simulink model "Final_Simulation_BMWi3_Average_Model"  (R2021b)
settings: Solver=FixedStepAuto  StartTime=0.0  StopTime=10  FixedStep=Tsim  RelTol=1e-3
values from neighbouring files (symbols this model uses):
  A_front = 2.38    [parameters_BMWi3.m]
  C_drag = 0.29    [parameters_BMWi3.m]
  flux_mach = 200/(6*4800*pi/30)    (= 0.0663145596216)    [parameters_BMWi3.m]
  fr = 0.013    [parameters_BMWi3.m]
  id = I_demand .* cos(beta)    [parameters_BMWi3.m]
  Imotor_max = 400    [parameters_BMWi3.m]
  iq = I_demand .* sin(beta)    [parameters_BMWi3.m]
  J_mach = 0.0666    [parameters_BMWi3.m]
  k_gear = nmax_mach/nmax_wheel    (= 5.46098838726)    [parameters_BMWi3.m]
  Ki_id = Bw_c^2 * Ld_mach    (= 846.812057613)    [parameters_BMWi3.m]
  Ki_idc = 2*pi*BW_i*R_Lboost    (= 471.238898038)    [parameters_BMWi3.m]
  Ki_iq = Bw_c^2 * Lq_mach    (= 2368.70505626)    [parameters_BMWi3.m]
  Ki_vdc = Wn_v^2*C_boost    (= 84.3851176293)    [parameters_BMWi3.m]
  Kp_id = 2*xi_c*Bw_c*Ld_mach-R_phase_mach    [parameters_BMWi3.m]
  Kp_idc = 2*pi*BW_i*L_boost    (= 1.88495559215)    [parameters_BMWi3.m]
  Kp_iq = 2*xi_c*Bw_c*Lq_mach-R_phase_mach    [parameters_BMWi3.m]
  Kp_vdc = 2*xi*Wn_v*C_boost    [parameters_BMWi3.m]
  Ld_mach = 0.0858*1e-3    (= 8.58e-05)    [parameters_BMWi3.m]
  Lq_mach = 0.24*1e-3    (= 0.00024)    [parameters_BMWi3.m]
  mass = 1270    [parameters_BMWi3.m]
  p = 6    [parameters_BMWi3.m]
  r_wheel = (15+2*70/(100*175))*0.0254/2    (= 0.1906016)    [parameters_BMWi3.m]
  rho = 1.25    [parameters_BMWi3.m]
  T = zeros(1,length(w))    [parameters_BMWi3.m]
  T_dq = (3/2)*(p)*(flux_mach*iq+(Ld_mach-Lq_mach)*iq.*id)    [parameters_BMWi3.m]
  Tmax_mach = 250    [parameters_BMWi3.m]
  Tsim = 5e-6    (= 5e-06)    [parameters_BMWi3.m]
  Vdc = 600    [parameters_BMWi3.m]
  w = 0:1:Wmax    [parameters_BMWi3.m]
  wbase = Pmax*1e3/Tmax    (= 500)    [parameters_BMWi3.m]
undefined symbols (not defined in the file or in its folder): Ion, Lithium
libraries: nesl_utility x18, fl_lib x14, spsSecondOrderFilterLib x10, sdl_lib x8, slpidlib x7, spsMeanLib x6, simulink x4, ee_lib x4, simulink_extras x3, pid_lib x2, spsabctodq0Lib x1, drivingcycle_lib x1
(part 2 of 2)

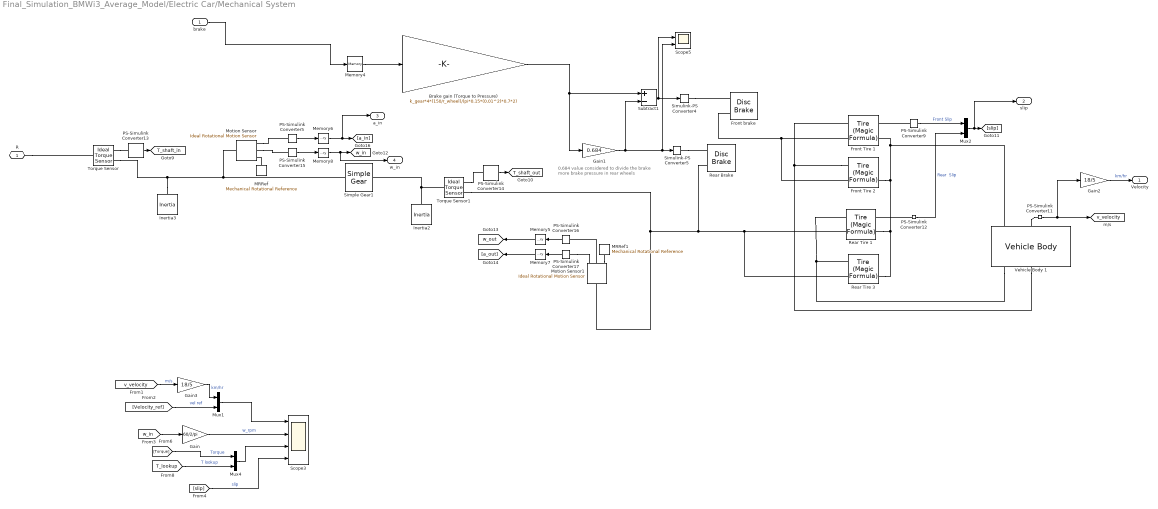
== system Final_Simulation_BMWi3_Average_Model/Electric Car/Mechanical System ==
  note: 0.684 value considered to divide the brake
      | more brake pressure in rear wheels
  brake : Inport
  " Rear Tire 1" : sdl_lib/Tires & Vehicles/Tire (Magic Formula)  parameterization=sdl.enum.magic_tire_model.peak  F_z1=3000 N  F_x1=3800 N  kappa1=10  B_m=10  C_m=1.9  D_m=1  E_m=0.97  fz0=4000 N  p_Cx=1.685  p_Dx=[1.21, -.037]  p_Ex=[.344, .095, -.02, 0]  p_Kx=[21.51, -.163, .245]  p_Hx=[-.002, .002]  p_Vx=[0, 0]  r_e=r_wheel m  model_compliance=sdl.enum.compliance.off  stiffness=1e6 N/m  damping=1000 N/(m/s)  model_inertia=sdl.enum.model_inertia.off  inertia=1 kg*m^2  initial_velocity=0 rad/s  model_resistance=simscape.enum.onoff.off  resistance_model=sdl.enum.rollingResistanceParameterization.velocity  coeff=0.015  p_tire=250e3 Pa  alpha=-0.003  beta=0.97  coeff_a=84e-4  coeff_b=6.2e-4 s/m  coeff_c=1.6e-4 s^2/m^2  v_thr=0.001 m/s  v_tr_thr=0.1 m/s
  Brake gain (Torque to Pressure) : Gain  Gain=k_gear*4*(150/r_wheel)/(pi*0.15*(0.01^2)*0.7*2)
  Front Tire 1 : sdl_lib/Tires & Vehicles/Tire (Magic Formula)  parameterization=sdl.enum.magic_tire_model.peak  F_z1=3000 N  F_x1=3800 N  kappa1=10  B_m=10  C_m=1.9  D_m=1  E_m=0.97  fz0=4000 N  p_Cx=1.685  p_Dx=[1.21, -.037]  p_Ex=[.344, .095, -.02, 0]  p_Kx=[21.51, -.163, .245]  p_Hx=[-.002, .002]  p_Vx=[0, 0]  r_e=r_wheel m  model_compliance=sdl.enum.compliance.off  stiffness=1e6 N/m  damping=1000 N/(m/s)  model_inertia=sdl.enum.model_inertia.off  inertia=1 kg*m^2  initial_velocity=0 rad/s  model_resistance=simscape.enum.onoff.off  resistance_model=sdl.enum.rollingResistanceParameterization.velocity  coeff=0.015  p_tire=250e3 Pa  alpha=-0.003  beta=0.97  coeff_a=84e-4  coeff_b=6.2e-4 s/m  coeff_c=1.6e-4 s^2/m^2  v_thr=0.001 m/s  v_tr_thr=0.1 m/s
  Front Tire 2 : sdl_lib/Tires & Vehicles/Tire (Magic Formula)  parameterization=sdl.enum.magic_tire_model.peak  F_z1=3000 N  F_x1=3800 N  kappa1=10  B_m=10  C_m=1.9  D_m=1  E_m=0.97  fz0=4000 N  p_Cx=1.685  p_Dx=[1.21, -.037]  p_Ex=[.344, .095, -.02, 0]  p_Kx=[21.51, -.163, .245]  p_Hx=[-.002, .002]  p_Vx=[0, 0]  r_e=r_wheel m  model_compliance=sdl.enum.compliance.off  stiffness=1e6 N/m  damping=1000 N/(m/s)  model_inertia=sdl.enum.model_inertia.off  inertia=1 kg*m^2  initial_velocity=0 rad/s  model_resistance=simscape.enum.onoff.off  resistance_model=sdl.enum.rollingResistanceParameterization.velocity  coeff=0.015  p_tire=250e3 Pa  alpha=-0.003  beta=0.97  coeff_a=84e-4  coeff_b=6.2e-4 s/m  coeff_c=1.6e-4 s^2/m^2  v_thr=0.001 m/s  v_tr_thr=0.1 m/s
  Front brake : sdl_lib/Brakes & Detents/Rotational/Disc Brake  r_mean=150 mm  bore=10 mm  n_pads=2  thermal_port=simscape.enum.thermaleffects.omit  mu_static=0.9  mu_coulomb=0.7  temperature_TLU=[280, 300, 320] K  mu_static_TLU=[.9, .8, .7]  mu_coulomb_TLU=[.8, .7, .6]  brkwy_vel=0.1 rad/s  visc_coef=.001 N*m/(rad/s)  enable_faults=simscape.enum.onoff.off  faulted_pressure=0 bar  external_fault=simscape.enum.onoff.off  temporal_fault=simscape.enum.onoff.off  fault_time=5 s  report_fault=simscape.enum.assert.action.none  thermal_mass=50 kJ/K  temperature_specify=off  temperature_priority=High  temperature=300 K  temperature_nominal_specify=off  temperature_nominal_unit=K  temperature_nominal_value=1
      settings: SourceProductBaseCode=LD
  Gain : Gain  Gain=60/2/pi
  Gain1 : Gain  Gain=0.684
  Gain2 : Gain  Gain=18/5
  Gain3 : Gain  Gain=18/5
  Inertia2 : fl_lib/Mechanical/Rotational Elements/Inertia  inertia=J_mach kg*m^2  num_ports=foundation.enum.numPorts2.one  w_specify=off  w_priority=High  w=0 rad/s  w_nominal_specify=off  w_nominal_unit=rad/s  w_nominal_value=1  t_specify=off  t_priority=None  t=0 N*m  t_nominal_specify=off  t_nominal_unit=N*m  t_nominal_value=1
  Inertia3 : fl_lib/Mechanical/Rotational Elements/Inertia  inertia=J_mach kg*m^2  num_ports=foundation.enum.numPorts2.one  w_specify=off  w_priority=High  w=0 rad/s  w_nominal_specify=off  w_nominal_unit=rad/s  w_nominal_value=1  t_specify=off  t_priority=None  t=0 N*m  t_nominal_specify=off  t_nominal_unit=N*m  t_nominal_value=1
  MRRef : fl_lib/Mechanical/Rotational Elements/Mechanical Rotational Reference
      settings: SourceProductName=Foundation Library
  MRRef1 : fl_lib/Mechanical/Rotational Elements/Mechanical Rotational Reference
      settings: SourceProductName=Foundation Library
  Memory{4..8} (5 alike) : Memory
  Motion Sensor : fl_lib/Mechanical/Mechanical Sensors/Ideal Rotational Motion Sensor  wrap_angle=simscape.enum.onoff.off  offset=0 rad
      settings: SourceProductName=Foundation Library
  Motion Sensor1 : fl_lib/Mechanical/Mechanical Sensors/Ideal Rotational Motion Sensor  wrap_angle=simscape.enum.onoff.off  offset=0 rad
      settings: SourceProductName=Foundation Library
  Mux1 : Mux  Inputs=2
  Mux2 : Mux  Inputs=2
  Mux4 : Mux  Inputs=2
  PS-Simulink Converter{5,9,11..12,15..17} (7 alike) : nesl_utility/PS-Simulink Converter  PhysicalDomain=network_engine_domain  SubClassName=ps_output  LeftPortType=input  RightPortType=output  PseudoPeriodic=off  Frequencies=[]  Unit=inherit  AffineConversion=off
      PS-Simulink Converter15 settings: SourceProductBaseCode=PW,SS
      PS-Simulink Converter16 settings: SourceProductBaseCode=PW,SS
      PS-Simulink Converter17 settings: SourceProductBaseCode=PW,SS
      PS-Simulink Converter5 settings: SourceProductBaseCode=PW,SS
  PS-Simulink Converter13 : nesl_utility/PS-Simulink Converter  PhysicalDomain=network_engine_domain  SubClassName=ps_output  LeftPortType=input  RightPortType=output  PseudoPeriodic=off  Frequencies=[]  Unit=N*m  AffineConversion=off
      settings: SourceProductName=Utilities
  PS-Simulink Converter14 : nesl_utility/PS-Simulink Converter  PhysicalDomain=network_engine_domain  SubClassName=ps_output  LeftPortType=input  RightPortType=output  PseudoPeriodic=off  Frequencies=[]  Unit=N*m  AffineConversion=off
      settings: SourceProductName=Utilities
  Rear Brake : sdl_lib/Brakes & Detents/Rotational/Disc Brake  r_mean=150 mm  bore=10 mm  n_pads=2  thermal_port=simscape.enum.thermaleffects.omit  mu_static=0.9  mu_coulomb=0.7  temperature_TLU=[280, 300, 320] K  mu_static_TLU=[.9, .8, .7]  mu_coulomb_TLU=[.8, .7, .6]  brkwy_vel=0.1 rad/s  visc_coef=.001 N*m/(rad/s)  enable_faults=simscape.enum.onoff.off  faulted_pressure=0 bar  external_fault=simscape.enum.onoff.off  temporal_fault=simscape.enum.onoff.off  fault_time=5 s  report_fault=simscape.enum.assert.action.none  thermal_mass=50 kJ/K  temperature_specify=off  temperature_priority=High  temperature=300 K  temperature_nominal_specify=off  temperature_nominal_unit=K  temperature_nominal_value=1
      settings: SourceProductBaseCode=LD
  Rear Tire 3 : sdl_lib/Tires & Vehicles/Tire (Magic Formula)  parameterization=sdl.enum.magic_tire_model.peak  F_z1=3000 N  F_x1=3800 N  kappa1=10  B_m=10  C_m=1.9  D_m=1  E_m=0.97  fz0=4000 N  p_Cx=1.685  p_Dx=[1.21, -.037]  p_Ex=[.344, .095, -.02, 0]  p_Kx=[21.51, -.163, .245]  p_Hx=[-.002, .002]  p_Vx=[0, 0]  r_e=r_wheel m  model_compliance=sdl.enum.compliance.off  stiffness=1e6 N/m  damping=1000 N/(m/s)  model_inertia=sdl.enum.model_inertia.off  inertia=1 kg*m^2  initial_velocity=0 rad/s  model_resistance=simscape.enum.onoff.off  resistance_model=sdl.enum.rollingResistanceParameterization.velocity  coeff=0.015  p_tire=250e3 Pa  alpha=-0.003  beta=0.97  coeff_a=84e-4  coeff_b=6.2e-4 s/m  coeff_c=1.6e-4 s^2/m^2  v_thr=0.001 m/s  v_tr_thr=0.1 m/s
  Scope3 : Scope  NumInputPorts=4
  Scope5 : Scope  NumInputPorts=2
  Simple Gear1 : sdl_lib/Gears/Simple Gear  ratio=k_gear  rotation_direction=sdl.enum.shaftOutputDirection.same  friction_model=sdl.enum.gear_efficiencies_load.off  T_noload=0.1 N*m  T_nom=5 N*m  efficiency_nom=0.8  efficiency=0.8  temperature_TLU=[280, 300, 320] K  load_TLU=[1, 5, 10] N*m  efficiency_TLU=[.95, .9, .85]  efficiency_TLU2=[.85, .8, .75; .95, .9, .85; .85, .8, .7]  w_thr=0.01 rad/s  pwr_thr=0.001 W  backlash_model=sdl.enum.backlashModel.Off  backlash_distance=1e-3 mm  x0=0 mm  r_base=0.1 m  hardstop_model=simscape.enum.hardstop.smooth  transition=1e-4 mm  backlash_stiffness=1e7 N/m  backlash_damping=1e6 N/(m/s)  e=0  v_tol=0.001 m/s  mu_visc=[0, 0] N*m/(rad/s)  enable_faults=simscape.enum.onoff.off  efficiency_fault=0.05  external_fault=simscape.enum.onoff.off  temporal_fault=simscape.enum.onoff.off  fault_time=5 s  fault_angles=pi / 12 rad  report_fault=simscape.enum.assert.action.none  thermal_mass=50 J/K  temperature_specify=off  temperature_priority=High  temperature=300 K  temperature_nominal_specify=off  temperature_nominal_unit=K  temperature_nominal_value=1  x_backlash_specify=off  x_backlash_priority=None  x_backlash=0 mm  x_backlash_nominal_specify=off  x_backlash_nominal_unit=mm  x_backlash_nominal_value=1  f_hardstop_specify=off  f_hardstop_priority=None  f_hardstop=0 N  f_hardstop_nominal_specify=off  f_hardstop_nominal_unit=N  f_hardstop_nominal_value=1  v_backlash_specify=off  v_backlash_priority=None  v_backlash=0 m/s  v_backlash_nominal_specify=off  v_backlash_nominal_unit=m/s  v_backlash_nominal_value=1
  Simulink-PS Converter4 : nesl_utility/Simulink-PS Converter  PhysicalDomain=network_engine_domain  SubClassName=ps_input  LeftPortType=input  RightPortType=output  PseudoPeriodic=off  Frequencies=[]  NoiseDistribution=none  NoiseParameters=[]  Unit=Pa  AffineConversion=off  FilteringAndDerivatives=provide  SimscapeFilterOrder=1  InputFilterTimeConstant=0.001  UdotUserProvided=0
  Simulink-PS Converter5 : nesl_utility/Simulink-PS Converter  PhysicalDomain=network_engine_domain  SubClassName=ps_input  LeftPortType=input  RightPortType=output  PseudoPeriodic=off  Frequencies=[]  NoiseDistribution=none  NoiseParameters=[]  Unit=Pa  AffineConversion=off  FilteringAndDerivatives=provide  SimscapeFilterOrder=1  InputFilterTimeConstant=0.001  UdotUserProvided=0
  Subtract1 : Sum  Inputs=+-
  Torque Sensor : fl_lib/Mechanical/Mechanical Sensors/Ideal Torque Sensor
      settings: SourceProductName=Foundation Library
  Torque Sensor1 : fl_lib/Mechanical/Mechanical Sensors/Ideal Torque Sensor
      settings: SourceProductName=Foundation Library
  Vehicle Body 1 : sdl_lib/Tires & Vehicles/Vehicle Body  mass=mass kg  n_w=2  x_f=1.2 m  x_r=1.37 m  y_c=CoG_z m  mass_var=simscape.enum.onoff.off  g=9.81 m/s^2  liftoff_warning=simscape.enum.onoff.off  area=A_front m^2  Cd=C_drag  rho=1.18 kg/m^3  model_pitch=simscape.enum.onoff.off  inertia=4000 kg*m^2  suspension_model=sdl.enum.linearTLU.linear  k_f=1e4 N/m  b_f=1e4 N/(m/s)  k_r=1e4 N/m  b_r=1e4 N/(m/s)  k_f_TLU=[-2000, -1000, 0, 1000, 2000] N  x_f_TLU=[-.4, -.2, 0, .2, .4] m  b_f_TLU=[-200, -100, 0, 100, 200] N  v_f_TLU=[-4, -2, 0, 2, 4] m/s  k_r_TLU=[-2000, -1000, 0, 1000, 2000] N  x_r_TLU=[-.4, -.2, 0, .2, .4] m  b_r_TLU=[-200, -100, 0, 100, 200] N  v_r_TLU=[-4, -2, 0, 2, 4] m/s  interp_method=simscape.enum.interpolation.linear  extrap_method=simscape.enum.extrapolation.linear  model_hardstop=simscape.enum.onoff.off  upper_bound_f=.25 m  lower_bound_f=-.25 m  stop_k_f=1e6 N/m  stop_b_f=150 N/(m/s)  upper_bound_r=.25 m  lower_bound_r=-.25 m  stop_k_r=1e6 N/m  stop_b_r=150 N/(m/s)  initial_pitch=0 rad  initial_pitch_rate=0 rad/s  v_specify=off  v_priority=High  v=0 m/s  v_nominal_specify=off  v_nominal_unit=m/s  v_nominal_value=1
  R : PMIOPort  Side=Left
  Velocity : Outport
  slip : Outport  Port=2
  a_in : Outport  Port=3
  w_in : Outport  Port=4
  tag scope: T_shaft_in=global, T_shaft_out=global, v_velocity=global, w_in=global, w_out=global
  wires:
  PS-Simulink Converter17/1 -> Memory7/1
  Memory8/1 -> w_in/1, [w_in]
  [w_in] -> Gain/1
  PS-Simulink Converter13/1 -> [T_shaft_in]
  [Velocity_ref] -> Mux1/2  "vel ref"
  PS-Simulink Converter16/1 -> Memory5/1
  PS-Simulink Converter9/1 -> Mux2/1  "Front Slip"
  PS-Simulink Converter5/1 -> Memory6/1
  Gain/1 -> Scope3/2  "w_rpm"
  PS-Simulink Converter15/1 -> Memory8/1
  Memory7/1 -> [a_out]
  Memory5/1 -> [w_out]
  [T_lookup] -> Mux4/2  "T lookup"
  Memory4/1 -> Brake gain (Torque to Pressure)/1
  Subtract1/1 -> Scope5/1, Simulink-PS Converter4/1
  Memory6/1 -> a_in/1, [a_in]
  Brake gain (Torque to Pressure)/1 -> Gain1/1, Subtract1/1
  Mux2/1 -> slip/1, [slip]
  [Torque] -> Mux4/1  "Torque"
  PS-Simulink Converter12/1 -> Mux2/2  "Rear  Slip"
  [v_velocity] -> Gain3/1  "m/s"
  [slip] -> Scope3/4  "slip"
  Gain1/1 -> Simulink-PS Converter5/1, Scope5/2, Subtract1/2
  Gain3/1 -> Mux1/1  "km/hr"
  PS-Simulink Converter14/1 -> [T_shaft_out]
  Mux4/1 -> Scope3/3
  Mux1/1 -> Scope3/1
  PS-Simulink Converter11/1 -> Gain2/1, [v_velocity]
  brake/1 -> Memory4/1
  Gain2/1 -> Velocity/1  "km/hr"
  connections:
  Front Tire 2/LConn1 -- Vehicle Body 1/RConn2 -- Front Tire 1/LConn1
  Front Tire 2/RConn2 -- Rear Tire 3/RConn2 -- " Rear Tire 1"/RConn2 -- Front Tire 1/RConn2 -- Vehicle Body 1/LConn1
  Motion Sensor1/LConn1 -- Rear Brake/LConn2 -- " Rear Tire 1"/LConn2 -- Rear Tire 3/LConn2 -- Torque Sensor1/RConn1
  Front Tire 1/LConn2 -- Front Tire 2/LConn2 -- Front brake/LConn2
  Torque Sensor1/LConn1 -- Inertia2/LConn1 -- Simple Gear1/RConn1
  " Rear Tire 1"/LConn1 -- Vehicle Body 1/RConn1 -- Rear Tire 3/LConn1
  Inertia3/LConn1 -- Simple Gear1/LConn1 -- Motion Sensor/LConn1 -- Torque Sensor/RConn1
  Motion Sensor1/RConn2 -- PS-Simulink Converter16/LConn1
  Motion Sensor/RConn2 -- PS-Simulink Converter15/LConn1
  PS-Simulink Converter17/LConn1 -- Motion Sensor1/RConn3
  MRRef/LConn1 -- Motion Sensor/RConn1
  Motion Sensor/RConn3 -- PS-Simulink Converter5/LConn1
  Simulink-PS Converter5/RConn1 -- Rear Brake/LConn1
  Torque Sensor1/RConn2 -- PS-Simulink Converter14/LConn1
  MRRef1/LConn1 -- Motion Sensor1/RConn1
  Torque Sensor/RConn2 -- PS-Simulink Converter13/LConn1
  Vehicle Body 1/LConn2 -- PS-Simulink Converter11/LConn1
  Simulink-PS Converter4/RConn1 -- Front brake/LConn1
  PS-Simulink Converter9/LConn1 -- Front Tire 1/RConn1
  PS-Simulink Converter12/LConn1 -- " Rear Tire 1"/RConn1
  R/RConn1 -- Torque Sensor/LConn1

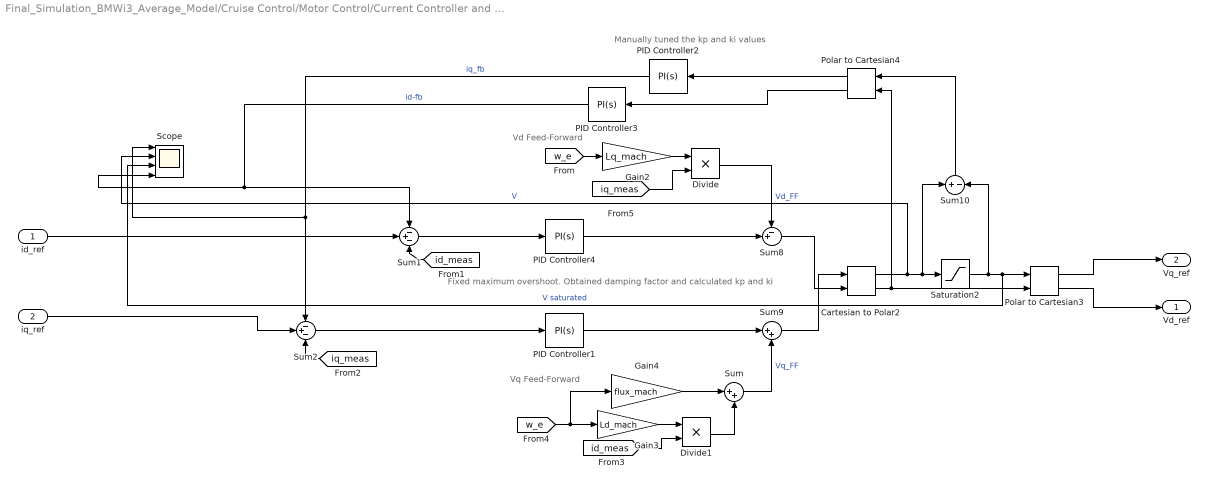
== system Final_Simulation_BMWi3_Average_Model/Cruise Control/Motor Control/Current Controller and Field Weakening ==
  note: Manually tuned the kp and ki values
  note: Fixed maximum overshoot. Obtained damping factor and calculated kp and ki
  note: Vd Feed-Forward
  note: Vq Feed-Forward
  id_ref : Inport
  iq_ref : Inport  Port=2
  Cartesian to Polar2 : simulink_extras/Transformations/Cartesian to Polar
  Divide : Product  Inputs=**
  Divide1 : Product  Inputs=**
  Gain2 : Gain  Gain=Lq_mach
  Gain3 : Gain  Gain=Ld_mach
  Gain4 : Gain  Gain=flux_mach
  PID Controller1 : slpidlib/PID Controller  Controller=PI  Form=Parallel  TimeDomain=Continuous-time  UseExternalTs=off  SampleTime=-1  IntegratorMethod=Forward Euler  FilterMethod=Forward Euler  ControllerParametersSource=internal  P=Kp_iq*1.4  I=Ki_iq*0.9  D=0  UseFilter=on  N=100  TunerSelectOption=Transfer Function Based (PID Tuner App)  InitialConditionSource=internal  InitialConditionForIntegrator=0  InitialConditionForFilter=0  DifferentiatorICPrevScaledInput=0  ExternalReset=none  TrackingMode=off  Kt=1  LimitOutput=on  SatLimitsSource=internal  UpperSaturationLimit=Vdc/sqrt(3)/sqrt(2)  LowerSaturationLimit=-Vdc/sqrt(3)/sqrt(2)  LinearizeAsGain=off  AntiWindupMode=clamping  Kb=1  POutMin=[]  POutMax=[]  IOutMin=[]  IOutMax=[]  DOutMin=[]  DOutMax=[]  NOutMin=[]  NOutMax=[]  SumOutMin=[]  SumOutMax=[]  SaturationOutMin=[]  SaturationOutMax=[]  PParamMin=[]  PParamMax=[]  IParamMin=[]  IParamMax=[]  DParamMin=[]  DParamMax=[]  NParamMin=[]  NParamMax=[]  KbParamMin=[]  KbParamMax=[]  KtParamMin=[]  KtParamMax=[]  KbOutMin=[]  KbOutMax=[]  KtOutMin=[]  KtOutMax=[]  IntegratorOutMin=[]  IntegratorOutMax=[]  FilterOutMin=[]  FilterOutMax=[]  SumI1OutMin=[]  SumI1OutMax=[]  SumI2OutMin=[]  SumI2OutMax=[]  SumI3OutMin=[]  SumI3OutMax=[]  SumI4OutMin=[]  SumI4OutMax=[]  SumDOutMin=[]  SumDOutMax=[]  DifferentiatorOutMin=[]  DifferentiatorOutMax=[]  FilterDiffOutCoefMin=[]  FilterDiffOutCoefMax=[]  ReciprocalOutMin=[]  ReciprocalOutMax=[]  SumDenOutMin=[]  SumDenOutMax=[]  SumNumOutMin=[]  SumNumOutMax=[]  DivideOutMin=[]  DivideOutMax=[]  UdiffTsProdOutMin=[]  UdiffTsProdOutMax=[]  NTsProdOutMin=[]  NTsProdOutMax=[]  UintegralTsProdOutMin=[]  UintegralTsProdOutMax=[]  UngainTsProdOutMin=[]  UngainTsProdOutMax=[]  IntegratorContinuousStateAttributes=''  IntegratorStateMustResolveToSignalObject=off  IntegratorRTWStateStorageClass=Auto  FilterContinuousStateAttributes=''  FilterStateMustResolveToSignalObject=off  FilterRTWStateStorageClass=Auto  ParallelPVariant=InternalParameters  IdealPVariant=Disabled  IVariant=InternalParameters  DVariant=Disabled  IntegratorVariant=Continuous  SatVariant=Enabled  AWVariant=ContClampingParallel  PCopyVariant=Disabled  TRVariant=Disabled  FdbkBlocksVariant=Forward  IdealPFdbkVariant=Disabled  SatFdbkVariant=Disabled  DerivativeFilterVariant=Disabled  NVariant=Disabled  NCopyVariant=Disabled_SignalSpec  FilterICVariant=Disabled  IntegratorICVariant=InternalICs  ExternalResetVariant=Disabled  TRSumVariant=Passthrough  SumFdbkVariant=Disabled  SumVariant=Sum_PI  TsampFilterVariant=InternalTs  TsampNgainVariant=Passthrough  TsampIntegralVariant=Passthrough  ExternalSaturationOutDataTypeStr=Inherit: Same as second input
  PID Controller2 : slpidlib/PID Controller  Controller=PI  Form=Parallel  TimeDomain=Continuous-time  UseExternalTs=off  SampleTime=-1  IntegratorMethod=Forward Euler  FilterMethod=Forward Euler  ControllerParametersSource=internal  P=0.8  I=75  D=0  UseFilter=on  N=100  TunerSelectOption=Transfer Function Based (PID Tuner App)  InitialConditionSource=internal  InitialConditionForIntegrator=0  InitialConditionForFilter=0  DifferentiatorICPrevScaledInput=0  ExternalReset=none  TrackingMode=off  Kt=1  LimitOutput=on  SatLimitsSource=internal  UpperSaturationLimit=Imotor_max  LowerSaturationLimit=-Imotor_max  LinearizeAsGain=on  AntiWindupMode=none  Kb=1  POutMin=[]  POutMax=[]  IOutMin=[]  IOutMax=[]  DOutMin=[]  DOutMax=[]  NOutMin=[]  NOutMax=[]  SumOutMin=[]  SumOutMax=[]  SaturationOutMin=[]  SaturationOutMax=[]  PParamMin=[]  PParamMax=[]  IParamMin=[]  IParamMax=[]  DParamMin=[]  DParamMax=[]  NParamMin=[]  NParamMax=[]  KbParamMin=[]  KbParamMax=[]  KtParamMin=[]  KtParamMax=[]  KbOutMin=[]  KbOutMax=[]  KtOutMin=[]  KtOutMax=[]  IntegratorOutMin=[]  IntegratorOutMax=[]  FilterOutMin=[]  FilterOutMax=[]  SumI1OutMin=[]  SumI1OutMax=[]  SumI2OutMin=[]  SumI2OutMax=[]  SumI3OutMin=[]  SumI3OutMax=[]  SumI4OutMin=[]  SumI4OutMax=[]  SumDOutMin=[]  SumDOutMax=[]  DifferentiatorOutMin=[]  DifferentiatorOutMax=[]  FilterDiffOutCoefMin=[]  FilterDiffOutCoefMax=[]  ReciprocalOutMin=[]  ReciprocalOutMax=[]  SumDenOutMin=[]  SumDenOutMax=[]  SumNumOutMin=[]  SumNumOutMax=[]  DivideOutMin=[]  DivideOutMax=[]  UdiffTsProdOutMin=[]  UdiffTsProdOutMax=[]  NTsProdOutMin=[]  NTsProdOutMax=[]  UintegralTsProdOutMin=[]  UintegralTsProdOutMax=[]  UngainTsProdOutMin=[]  UngainTsProdOutMax=[]  IntegratorContinuousStateAttributes=''  IntegratorStateMustResolveToSignalObject=off  IntegratorRTWStateStorageClass=Auto  FilterContinuousStateAttributes=''  FilterStateMustResolveToSignalObject=off  FilterRTWStateStorageClass=Auto  ParallelPVariant=InternalParameters  IdealPVariant=Disabled  IVariant=InternalParameters  DVariant=Disabled  IntegratorVariant=Continuous  SatVariant=Enabled  AWVariant=Passthrough  PCopyVariant=Disabled  TRVariant=Disabled  FdbkBlocksVariant=Forward  IdealPFdbkVariant=Disabled  SatFdbkVariant=Disabled  DerivativeFilterVariant=Disabled  NVariant=Disabled  NCopyVariant=Disabled_SignalSpec  FilterICVariant=Disabled  IntegratorICVariant=InternalICs  ExternalResetVariant=Disabled  TRSumVariant=Passthrough  SumFdbkVariant=Disabled  SumVariant=Sum_PI  TsampFilterVariant=InternalTs  TsampNgainVariant=Passthrough  TsampIntegralVariant=Passthrough  ExternalSaturationOutDataTypeStr=Inherit: Same as second input
  PID Controller3 : slpidlib/PID Controller  Controller=PI  Form=Parallel  TimeDomain=Continuous-time  UseExternalTs=off  SampleTime=-1  IntegratorMethod=Forward Euler  FilterMethod=Forward Euler  ControllerParametersSource=internal  P=0.9  I=-10  D=0  UseFilter=on  N=100  TunerSelectOption=Transfer Function Based (PID Tuner App)  InitialConditionSource=internal  InitialConditionForIntegrator=0  InitialConditionForFilter=0  DifferentiatorICPrevScaledInput=0  ExternalReset=none  TrackingMode=off  Kt=1  LimitOutput=on  SatLimitsSource=internal  UpperSaturationLimit=Imotor_max/4  LowerSaturationLimit=-Imotor_max/4  LinearizeAsGain=on  AntiWindupMode=none  Kb=1  POutMin=[]  POutMax=[]  IOutMin=[]  IOutMax=[]  DOutMin=[]  DOutMax=[]  NOutMin=[]  NOutMax=[]  SumOutMin=[]  SumOutMax=[]  SaturationOutMin=[]  SaturationOutMax=[]  PParamMin=[]  PParamMax=[]  IParamMin=[]  IParamMax=[]  DParamMin=[]  DParamMax=[]  NParamMin=[]  NParamMax=[]  KbParamMin=[]  KbParamMax=[]  KtParamMin=[]  KtParamMax=[]  KbOutMin=[]  KbOutMax=[]  KtOutMin=[]  KtOutMax=[]  IntegratorOutMin=[]  IntegratorOutMax=[]  FilterOutMin=[]  FilterOutMax=[]  SumI1OutMin=[]  SumI1OutMax=[]  SumI2OutMin=[]  SumI2OutMax=[]  SumI3OutMin=[]  SumI3OutMax=[]  SumI4OutMin=[]  SumI4OutMax=[]  SumDOutMin=[]  SumDOutMax=[]  DifferentiatorOutMin=[]  DifferentiatorOutMax=[]  FilterDiffOutCoefMin=[]  FilterDiffOutCoefMax=[]  ReciprocalOutMin=[]  ReciprocalOutMax=[]  SumDenOutMin=[]  SumDenOutMax=[]  SumNumOutMin=[]  SumNumOutMax=[]  DivideOutMin=[]  DivideOutMax=[]  UdiffTsProdOutMin=[]  UdiffTsProdOutMax=[]  NTsProdOutMin=[]  NTsProdOutMax=[]  UintegralTsProdOutMin=[]  UintegralTsProdOutMax=[]  UngainTsProdOutMin=[]  UngainTsProdOutMax=[]  IntegratorContinuousStateAttributes=''  IntegratorStateMustResolveToSignalObject=off  IntegratorRTWStateStorageClass=Auto  FilterContinuousStateAttributes=''  FilterStateMustResolveToSignalObject=off  FilterRTWStateStorageClass=Auto  ParallelPVariant=InternalParameters  IdealPVariant=Disabled  IVariant=InternalParameters  DVariant=Disabled  IntegratorVariant=Continuous  SatVariant=Enabled  AWVariant=Passthrough  PCopyVariant=Disabled  TRVariant=Disabled  FdbkBlocksVariant=Forward  IdealPFdbkVariant=Disabled  SatFdbkVariant=Disabled  DerivativeFilterVariant=Disabled  NVariant=Disabled  NCopyVariant=Disabled_SignalSpec  FilterICVariant=Disabled  IntegratorICVariant=InternalICs  ExternalResetVariant=Disabled  TRSumVariant=Passthrough  SumFdbkVariant=Disabled  SumVariant=Sum_PI  TsampFilterVariant=InternalTs  TsampNgainVariant=Passthrough  TsampIntegralVariant=Passthrough  ExternalSaturationOutDataTypeStr=Inherit: Same as second input
  PID Controller4 : slpidlib/PID Controller  Controller=PI  Form=Parallel  TimeDomain=Continuous-time  UseExternalTs=off  SampleTime=-1  IntegratorMethod=Forward Euler  FilterMethod=Forward Euler  ControllerParametersSource=internal  P=Kp_id*1.3  I=Ki_id*0.9  D=0  UseFilter=on  N=100  TunerSelectOption=Transfer Function Based (PID Tuner App)  InitialConditionSource=internal  InitialConditionForIntegrator=0  InitialConditionForFilter=0  DifferentiatorICPrevScaledInput=0  ExternalReset=none  TrackingMode=off  Kt=1  LimitOutput=on  SatLimitsSource=internal  UpperSaturationLimit=Vdc/sqrt(3)/sqrt(2)  LowerSaturationLimit=-Vdc/sqrt(3)/sqrt(2)  LinearizeAsGain=off  AntiWindupMode=clamping  Kb=1  POutMin=[]  POutMax=[]  IOutMin=[]  IOutMax=[]  DOutMin=[]  DOutMax=[]  NOutMin=[]  NOutMax=[]  SumOutMin=[]  SumOutMax=[]  SaturationOutMin=[]  SaturationOutMax=[]  PParamMin=[]  PParamMax=[]  IParamMin=[]  IParamMax=[]  DParamMin=[]  DParamMax=[]  NParamMin=[]  NParamMax=[]  KbParamMin=[]  KbParamMax=[]  KtParamMin=[]  KtParamMax=[]  KbOutMin=[]  KbOutMax=[]  KtOutMin=[]  KtOutMax=[]  IntegratorOutMin=[]  IntegratorOutMax=[]  FilterOutMin=[]  FilterOutMax=[]  SumI1OutMin=[]  SumI1OutMax=[]  SumI2OutMin=[]  SumI2OutMax=[]  SumI3OutMin=[]  SumI3OutMax=[]  SumI4OutMin=[]  SumI4OutMax=[]  SumDOutMin=[]  SumDOutMax=[]  DifferentiatorOutMin=[]  DifferentiatorOutMax=[]  FilterDiffOutCoefMin=[]  FilterDiffOutCoefMax=[]  ReciprocalOutMin=[]  ReciprocalOutMax=[]  SumDenOutMin=[]  SumDenOutMax=[]  SumNumOutMin=[]  SumNumOutMax=[]  DivideOutMin=[]  DivideOutMax=[]  UdiffTsProdOutMin=[]  UdiffTsProdOutMax=[]  NTsProdOutMin=[]  NTsProdOutMax=[]  UintegralTsProdOutMin=[]  UintegralTsProdOutMax=[]  UngainTsProdOutMin=[]  UngainTsProdOutMax=[]  IntegratorContinuousStateAttributes=''  IntegratorStateMustResolveToSignalObject=off  IntegratorRTWStateStorageClass=Auto  FilterContinuousStateAttributes=''  FilterStateMustResolveToSignalObject=off  FilterRTWStateStorageClass=Auto  ParallelPVariant=InternalParameters  IdealPVariant=Disabled  IVariant=InternalParameters  DVariant=Disabled  IntegratorVariant=Continuous  SatVariant=Enabled  AWVariant=ContClampingParallel  PCopyVariant=Disabled  TRVariant=Disabled  FdbkBlocksVariant=Forward  IdealPFdbkVariant=Disabled  SatFdbkVariant=Disabled  DerivativeFilterVariant=Disabled  NVariant=Disabled  NCopyVariant=Disabled_SignalSpec  FilterICVariant=Disabled  IntegratorICVariant=InternalICs  ExternalResetVariant=Disabled  TRSumVariant=Passthrough  SumFdbkVariant=Disabled  SumVariant=Sum_PI  TsampFilterVariant=InternalTs  TsampNgainVariant=Passthrough  TsampIntegralVariant=Passthrough  ExternalSaturationOutDataTypeStr=Inherit: Same as second input
  Polar to Cartesian3 : simulink_extras/Transformations/Polar to Cartesian
      settings: SourceProductBaseCode=SL
  Polar to Cartesian4 : simulink_extras/Transformations/Polar to Cartesian
      settings: SourceProductBaseCode=SL
  Saturation2 : Saturate  UpperLimit=Vdc/sqrt(3)/sqrt(2)  LowerLimit=0
  Scope : Scope  NumInputPorts=4
  Sum : Sum  Inputs=|++
  Sum1 : Sum  Inputs=-+-
  Sum10 : Sum  Inputs=+|-
  Sum2 : Sum  Inputs=-+-
  Sum8 : Sum  Inputs=-+|
  Sum9 : Sum  Inputs=|++
  Vd_ref : Outport  VectorParamsAs1DForOutWhenUnconnected=off
  Vq_ref : Outport  Port=2  VectorParamsAs1DForOutWhenUnconnected=off
  wires:
  Polar to Cartesian3/2 -> Vd_ref/1
  Polar to Cartesian3/1 -> Vq_ref/1
  Sum1/1 -> PID Controller4/1
  PID Controller4/1 -> Sum8/2
  Sum2/1 -> PID Controller1/1
  PID Controller1/1 -> Sum9/1
  [w_e] -> Gain2/1
  Gain2/1 -> Divide/1
  [id_meas] -> Sum1/3
  [iq_meas] -> Sum2/3
  Divide/1 -> Sum8/1  "Vd_FF"
  [w_e] -> Gain4/1, Gain3/1
  Gain3/1 -> Divide1/1
  Gain4/1 -> Sum/1
  Divide1/1 -> Sum/2
  Sum/1 -> Sum9/2  "Vq_FF"
  Cartesian to Polar2/1 -> Scope/2, Sum10/1, Saturation2/1  "V"
  Cartesian to Polar2/2 -> Polar to Cartesian4/2, Polar to Cartesian3/2
  Saturation2/1 -> Sum10/2, Scope/3, Polar to Cartesian3/1  "V saturated"
  PID Controller2/1 -> Scope/1, Sum2/1  "iq_fb"
  Sum8/1 -> Cartesian to Polar2/2
  Sum9/1 -> Cartesian to Polar2/1
  Sum10/1 -> Polar to Cartesian4/1
  Polar to Cartesian4/1 -> PID Controller2/1
  Polar to Cartesian4/2 -> PID Controller3/1
  id_ref/1 -> Sum1/2
  iq_ref/1 -> Sum2/2
  [iq_meas] -> Divide/2
  [id_meas] -> Divide1/2
  PID Controller3/1 -> Sum1/1, Scope/4  "id-fb"

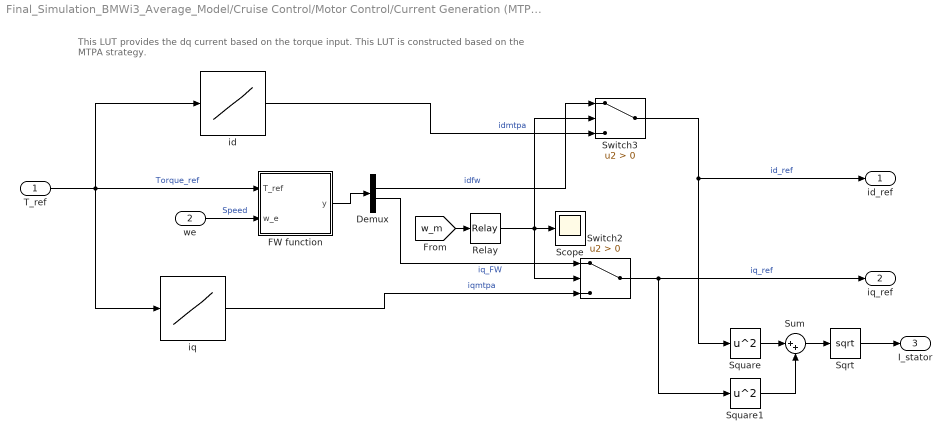
== system Final_Simulation_BMWi3_Average_Model/Cruise Control/Motor Control/Current Generation (MTPA) ==
  note: This LUT provides the dq current based on the torque input. This LUT is constructed based on the MTPA strategy.
  T_ref : Inport
  we : Inport  Port=2
  Demux : Demux
  "FW function " : MATLAB Function  TreatAsAtomicUnit=on
  Relay : Relay  OnSwitchValue=wbase+11400  OffSwitchValue=wbase-50
  Scope : Scope
  Sqrt : Sqrt  SaturateOnIntegerOverflow=on
  Square : Math  Operator=square  SaturateOnIntegerOverflow=on
  Square1 : Math  Operator=square  SaturateOnIntegerOverflow=on
  Sum : Sum  Inputs=|++
  Switch2 : Switch  Criteria=u2 > Threshold
  Switch3 : Switch  Criteria=u2 > Threshold
  id : Lookup_n-D  NumberOfTableDimensions=1  BreakpointsForDimension1=T_dq  Table=id  InterpMethod=Linear Lagrange  InternalRulePriority=Speed  RndMeth=Simplest  InputSameDT=on
  iq : Lookup_n-D  NumberOfTableDimensions=1  BreakpointsForDimension1=T_dq  Table=iq  InterpMethod=Linear Lagrange  InternalRulePriority=Speed  RndMeth=Simplest  InputSameDT=on
  id_ref : Outport  VectorParamsAs1DForOutWhenUnconnected=off
  iq_ref : Outport  Port=2  VectorParamsAs1DForOutWhenUnconnected=off
  I_stator : Outport  Port=3  VectorParamsAs1DForOutWhenUnconnected=off
  wires:
  "FW function "/1(y) -> Demux/1
  Switch2/1 -> iq_ref/1, Square1/1  "iq_ref"
  Switch3/1 -> Square/1, id_ref/1  "id_ref"
  we/1 -> "FW function "/2(w_e)  "Speed"
  id/1 -> Switch3/3  "idmtpa"
  iq/1 -> Switch2/3  "iqmtpa"
  T_ref/1 -> iq/1, id/1, "FW function "/1(T_ref)  "Torque_ref"
  Demux/2 -> Switch3/1  "idfw"
  Demux/3 -> Switch2/1  "iq_FW"
  Square/1 -> Sum/1
  Square1/1 -> Sum/2
  Sum/1 -> Sqrt/1
  Sqrt/1 -> I_stator/1
  Relay/1 -> Switch2/2, Switch3/2, Scope/1
  [w_m] -> Relay/1

== system Final_Simulation_BMWi3_Average_Model/Cruise Control/Torque Sharing/Enabled Subsystem ==
  Enable : EnablePort  StatesWhenEnabling=reset  PropagateVarSize=During execution
  Constant : Constant
  Sum1 : Sum  Inputs=|++  InputSameDT=on  SaturateOnIntegerOverflow=on  OutDataTypeStr=Inherit: Same as first input
  Unit Delay : UnitDelay  SampleTime=0.01  HasFrameUpgradeWarning=on
  eOut : Outport  InitialOutput=0  VectorParamsAs1DForOutWhenUnconnected=off
  wires:
  Sum1/1 -> Unit Delay/1
  Constant/1 -> Sum1/1
  Unit Delay/1 -> eOut/1, Sum1/2

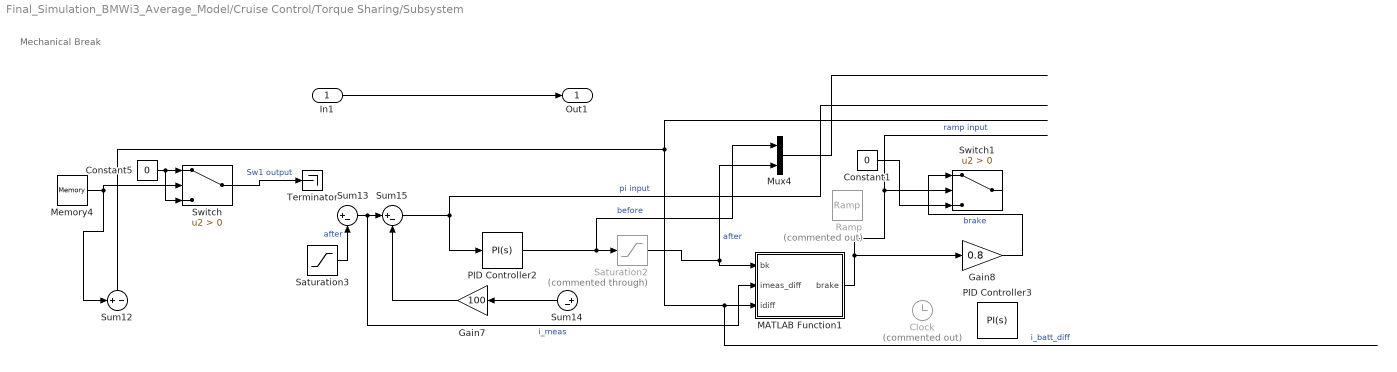
== system Final_Simulation_BMWi3_Average_Model/Cruise Control/Torque Sharing/Subsystem ==
  note: Mechanical Break
  In1 : Inport
  Clock : Clock  Commented=on
  Constant1 : Constant  Value=0
  Constant5 : Constant  Value=0
  Gain7 : Gain  Gain=100
  Gain8 : Gain  Gain=0.8
  MATLAB Function1 : MATLAB Function  TreatAsAtomicUnit=on
  Memory4 : Memory
  Mux4 : Mux  Inputs=2
  PID Controller2 : pid_lib/PID Controller  Controller=PI  Form=Parallel  TimeDomain=Continuous-time  UseExternalTs=off  SampleTime=-1  IntegratorMethod=Forward Euler  FilterMethod=Forward Euler  ControllerParametersSource=internal  P=10  I=0.1  D=0  UseFilter=on  N=100  TunerSelectOption=Transfer Function Based (PID Tuner App)  InitialConditionSource=internal  InitialConditionForIntegrator=0  InitialConditionForFilter=0  DifferentiatorICPrevScaledInput=0  ExternalReset=none  TrackingMode=off  Kt=1  LimitOutput=off  SatLimitsSource=internal  UpperSaturationLimit=150  LowerSaturationLimit=-150  LinearizeAsGain=off  AntiWindupMode=none  Kb=1  POutMin=[]  POutMax=[]  IOutMin=[]  IOutMax=[]  DOutMin=[]  DOutMax=[]  NOutMin=[]  NOutMax=[]  SumOutMin=[]  SumOutMax=[]  SaturationOutMin=[]  SaturationOutMax=[]  PParamMin=[]  PParamMax=[]  IParamMin=[]  IParamMax=[]  DParamMin=[]  DParamMax=[]  NParamMin=[]  NParamMax=[]  KbParamMin=[]  KbParamMax=[]  KtParamMin=[]  KtParamMax=[]  KbOutMin=[]  KbOutMax=[]  KtOutMin=[]  KtOutMax=[]  IntegratorOutMin=[]  IntegratorOutMax=[]  FilterOutMin=[]  FilterOutMax=[]  SumI1OutMin=[]  SumI1OutMax=[]  SumI2OutMin=[]  SumI2OutMax=[]  SumI3OutMin=[]  SumI3OutMax=[]  SumI4OutMin=[]  SumI4OutMax=[]  SumDOutMin=[]  SumDOutMax=[]  DifferentiatorOutMin=[]  DifferentiatorOutMax=[]  FilterDiffOutCoefMin=[]  FilterDiffOutCoefMax=[]  ReciprocalOutMin=[]  ReciprocalOutMax=[]  SumDenOutMin=[]  SumDenOutMax=[]  SumNumOutMin=[]  SumNumOutMax=[]  DivideOutMin=[]  DivideOutMax=[]  UdiffTsProdOutMin=[]  UdiffTsProdOutMax=[]  NTsProdOutMin=[]  NTsProdOutMax=[]  UintegralTsProdOutMin=[]  UintegralTsProdOutMax=[]  UngainTsProdOutMin=[]  UngainTsProdOutMax=[]  IntegratorContinuousStateAttributes=''  IntegratorStateMustResolveToSignalObject=off  IntegratorRTWStateStorageClass=Auto  FilterContinuousStateAttributes=''  FilterStateMustResolveToSignalObject=off  FilterRTWStateStorageClass=Auto  ParallelPVariant=InternalParameters  IdealPVariant=Disabled  IVariant=InternalParameters  DVariant=Disabled  IntegratorVariant=Continuous  SatVariant=Disabled  AWVariant=Passthrough  PCopyVariant=Disabled  TRVariant=Disabled  FdbkBlocksVariant=Forward  IdealPFdbkVariant=Disabled  SatFdbkVariant=Disabled  DerivativeFilterVariant=Disabled  NVariant=Disabled  NCopyVariant=Disabled_SignalSpec  FilterICVariant=Disabled  IntegratorICVariant=InternalICs  ExternalResetVariant=Disabled  TRSumVariant=Passthrough  SumFdbkVariant=Disabled  SumVariant=Sum_PI  TsampFilterVariant=InternalTs  TsampNgainVariant=Passthrough  TsampIntegralVariant=Passthrough  ExternalSaturationOutDataTypeStr=Inherit: Same as second input
  PID Controller3 : pid_lib/PID Controller  Controller=PI  Form=Parallel  TimeDomain=Continuous-time  UseExternalTs=off  SampleTime=-1  IntegratorMethod=Forward Euler  FilterMethod=Forward Euler  ControllerParametersSource=internal  P=0.01  I=100  D=0  UseFilter=on  N=100  TunerSelectOption=Transfer Function Based (PID Tuner App)  InitialConditionSource=internal  InitialConditionForIntegrator=0  InitialConditionForFilter=0  DifferentiatorICPrevScaledInput=0  ExternalReset=none  TrackingMode=off  Kt=1  LimitOutput=off  SatLimitsSource=internal  UpperSaturationLimit=inf  LowerSaturationLimit=-inf  LinearizeAsGain=on  AntiWindupMode=none  Kb=1  POutMin=[]  POutMax=[]  IOutMin=[]  IOutMax=[]  DOutMin=[]  DOutMax=[]  NOutMin=[]  NOutMax=[]  SumOutMin=[]  SumOutMax=[]  SaturationOutMin=[]  SaturationOutMax=[]  PParamMin=[]  PParamMax=[]  IParamMin=[]  IParamMax=[]  DParamMin=[]  DParamMax=[]  NParamMin=[]  NParamMax=[]  KbParamMin=[]  KbParamMax=[]  KtParamMin=[]  KtParamMax=[]  KbOutMin=[]  KbOutMax=[]  KtOutMin=[]  KtOutMax=[]  IntegratorOutMin=[]  IntegratorOutMax=[]  FilterOutMin=[]  FilterOutMax=[]  SumI1OutMin=[]  SumI1OutMax=[]  SumI2OutMin=[]  SumI2OutMax=[]  SumI3OutMin=[]  SumI3OutMax=[]  SumI4OutMin=[]  SumI4OutMax=[]  SumDOutMin=[]  SumDOutMax=[]  DifferentiatorOutMin=[]  DifferentiatorOutMax=[]  FilterDiffOutCoefMin=[]  FilterDiffOutCoefMax=[]  ReciprocalOutMin=[]  ReciprocalOutMax=[]  SumDenOutMin=[]  SumDenOutMax=[]  SumNumOutMin=[]  SumNumOutMax=[]  DivideOutMin=[]  DivideOutMax=[]  UdiffTsProdOutMin=[]  UdiffTsProdOutMax=[]  NTsProdOutMin=[]  NTsProdOutMax=[]  UintegralTsProdOutMin=[]  UintegralTsProdOutMax=[]  UngainTsProdOutMin=[]  UngainTsProdOutMax=[]  IntegratorContinuousStateAttributes=''  IntegratorStateMustResolveToSignalObject=off  IntegratorRTWStateStorageClass=Auto  FilterContinuousStateAttributes=''  FilterStateMustResolveToSignalObject=off  FilterRTWStateStorageClass=Auto  ParallelPVariant=InternalParameters  IdealPVariant=Disabled  IVariant=InternalParameters  DVariant=Disabled  IntegratorVariant=Continuous  SatVariant=Disabled  AWVariant=Passthrough  PCopyVariant=Disabled  TRVariant=Disabled  FdbkBlocksVariant=Forward  IdealPFdbkVariant=Disabled  SatFdbkVariant=Disabled  DerivativeFilterVariant=Disabled  NVariant=Disabled  NCopyVariant=Disabled_SignalSpec  FilterICVariant=Disabled  IntegratorICVariant=InternalICs  ExternalResetVariant=Disabled  TRSumVariant=Passthrough  SumFdbkVariant=Disabled  SumVariant=Sum_PI  TsampFilterVariant=InternalTs  TsampNgainVariant=Passthrough  TsampIntegralVariant=Passthrough  ExternalSaturationOutDataTypeStr=Inherit: Same as second input
  Ramp : simulink/Sources/Ramp  Commented=on  slope=0.01  start=0  InitialOutput=0
  Saturation2 : Saturate  Commented=through  UpperLimit=0.25  LowerLimit=-0.25
  Saturation3 : Saturate  UpperLimit=352  LowerLimit=-352
  Sum12 : Sum  Inputs=+-
  Sum13 : Sum  Inputs=|+-
  Sum14 : Sum  Inputs=|+-
  Sum15 : Sum  Inputs=|+-
  Switch : Switch  Criteria=u2 > Threshold
  Switch1 : Switch  Criteria=u2 > Threshold
  Terminator : Terminator
  Out1 : Outport
  wires:
  In1/1 -> Out1/1
  ? -> ?  "ramp input"
  Sum12/1 -> MATLAB Function1/3(idiff)  "i_batt_diff"
  ? -> ?
  Gain7/1 -> Sum15/2
  ? -> Saturation3/1, Sum13/1
  Sum14/1 -> Gain7/1
  PID Controller2/1 -> Saturation2/1, Mux4/1  "before"
  ? -> ?
  Constant5/1 -> Switch/3, Switch/1
  Switch/1 -> Terminator/1  "Sw1 output"
  ? -> Memory4/1
  Saturation2/1 -> Mux4/2, MATLAB Function1/1(bk)  "after"
  MATLAB Function1/1(brake) -> Gain8/1, Switch1/2  "ramp input"
  Constant1/1 -> Switch1/3
  Sum15/1 -> PID Controller2/1  "pi input"
  Sum13/1 -> MATLAB Function1/2(imeas_diff), Sum15/1  "i_meas"
  Memory4/1 -> Sum12/1, Switch/2
  ? -> ?
  Gain8/1 -> Switch1/1  "brake"
  ? -> Sum12/2
  Saturation3/1 -> Sum13/2  "after"
  Mux4/1 -> ?

== matlab function Final_Simulation_BMWi3_Average_Model/Cruise Control/Motor Control/Current Generation (MTPA)/FW function  ==
  data: T_ref input; y output; w_e input
function y = fcn(T_ref, w_e)

Vdc = 600;
Lq = 0.24*1e-3;
Ld = 0.0858*1e-3;
phi_m = 200/(6*4800*pi/30);
T_max = 250;
p = 6;
w_b = 500;
Imotor_max = 400;
w_m = w_e/p;

% Lq, Ld, p, phi_m, Vdc, wb,T_max,
Vmax = Vdc/sqrt(3); % maximum line to neutral voltage
% MTPA
T = max(T_ref, T_max); % Limiting the torque
Im = 2*T/(3*p*phi_m); % estimated max current
Im = max(Imotor_max, Im);
a = Ld-Lq;            % constant 1
b = Ld^2-Lq^2;        % constant 2
c = Vmax^2/w_e^2;     % constant 3
id_mtpa = (phi_m/4*a)-sqrt((phi_m^2/(16*a^2))+(Im^2/2)); % d-axis phase current MTPA table
iq_mtpa = sqrt(Im^2-id_mtpa^2);                          % q-axis phase current MTPA table
% % 
% I_step = 0.05;    % [A]
% I_demand = -Imotor_max: I_step : Imotor_max;      
% beta = acos((-phi_m + sqrt(phi_m^2 + 8* (Ld-Lq)^2 * I_demand.^2)) ./ (4*(Ld-Lq)*I_demand));
% id = I_demand .* cos(beta);
% iq = I_demand .* sin(beta);
% % plot(sqrt(id(p)^2+iq(p)^2),Tdq);
% T_dq = (3/2)*(p)*(phi_m*iq+(Ld-Lq)*iq.*id); % Mechanical torque in rotor frame (not rotor flux) as required by simulink

% idmtpa = fixpt_interp1(id,T_dq,279,2^-3,sfix(8), 2^-3,sfix(16),'Floor')
% iqmtpa = fixpt_interp1(iq,T_dq,279,2^-3, 2^-3,'Floor')

% Flux Weakening
imax = Imotor_max; % maximum motor current
k1 = ((phi_m*Ld)^2-(b*(phi_m^2+(Lq*imax)^2-c)));
if k1<0
    k = 0;
else
    k = k1;
end
% k=k1;
id_fw = ((-phi_m*Ld)+sqrt(k))/(b);  % d-axis flux weakening current

idfw = max(id_fw, -imax);    % d-axis flux weakening current with limitation 
iqfw = sqrt(imax^2-idfw^2);   % q-axis flux weakening current
T_fw = (3*p/2)*((phi_m*iqfw)+(a*idfw*iqfw)); % Flux weakening torque
 

id_ref =0;
iq_ref = 0;
iq_ref1 =0;
% current command selection based on the speed and torque ref
if (abs(w_m) < w_b)
    
     id_ref = id_mtpa;
     iq_ref = iq_mtpa;
    
else
if (abs(w_m) > w_b)
     if (T_fw < T_ref)
         id_ref = idfw;
         iq_ref = iqfw;

     else
         id_ref = idfw;
         iq_ref = T_ref/((3*p/2)*(phi_m+(a*idfw)));
         iq_ref1 = T_ref/((3*p/2)*(phi_m+(a*idfw)));
     end
end
end
i = sqrt(id_ref.^2+iq_ref.^2);
y = [i, id_ref, iq_ref,iq_ref1];

== matlab function Final_Simulation_BMWi3_Average_Model/Cruise Control/Torque Sharing/Subsystem/MATLAB Function1 ==
  data: bk input; brake output; imeas_diff input; idiff input
function brake   = fcn(bk, imeas_diff, idiff)
brake = 0;
count = 0;
if imeas_diff>5
  brake = bk;
elseif idiff>0
    brake = bk;
else
    brake = 0;
    count = 0;
end

== matlab function Final_Simulation_BMWi3_Average_Model/Cruise Control/Torque Sharing/Torque_Sharing ==
  data: brake output; Tref input; i_meas_diff input; ibatt_diff input; Tref_out output; SOC input; test output
% function [brake, Tref_out,test] = fcn( Tref, i_meas_diff, ibatt_diff, SOC)
%  brake = 0;
%  Tref_out = 0;
%  test =0;
%  coder.extrinsic('Torque_Sharing');
%  [brake, Tref_out,test] = Torque_Sharing(Tref, i_meas_diff, ibatt_diff, SOC);
% end
function [brake, Tref_out, test] = fcn(Tref, i_meas_diff, ibatt_diff, SOC)
brake = 0;
Tref_out = Tref;
test = 10;
if SOC<=80
     if (Tref<0 || (i_meas_diff>100 &&i_meas_diff>80) )
     Tref_out = Tref./5;
     brake = 0.3;
     test = 1;
     elseif (Tref<0 || (i_meas_diff>80 && i_meas_diff<60)|| ibatt_diff>5)
     Tref_out = Tref./4;
     brake = 0.28;  
     test = 2;
     elseif (Tref<0 || (i_meas_diff>60 && i_meas_diff>40) || ibatt_diff>5)
     Tref_out = Tref./3;
     brake = 0.25;  
     test = 3;
     elseif (Tref<0 || (i_meas_diff>40 && i_meas_diff<20) || ibatt_diff>5)
     Tref_out = Tref./2;
     brake = 0.2;  
     test = 4;
     elseif (Tref<0 || i_meas_diff>20 || ibatt_diff>5)
     Tref_out = Tref./2;
     brake = 0.18; 
     test = 5;
     else
     Tref_out = Tref;
     brake = 0;
     test =6;
    end
 end
 if (SOC>80 || Tref<0 || i_meas_diff>2)
      Tref_out = 0;
      brake = 0.2;
      test =7;
%  else
%      Tref_out = Tref;
%      brake = 0;
%      test=6;
 end
%[brake, Tref_out,test] = Torque_Sharing(Tref, i_meas_diff, ibatt_diff, SOC);         
end

== matlab function Final_Simulation_BMWi3_Average_Model/Electric Car/Battery/MATLAB Function ==
  data: SOC input; Ibmax output; Ibmin output
function [Ibmax,Ibmin]  = fcn(SOC)
Imax = 400;
Imin = -100;
Ibmax = Imax;
Ibmin = Imin;
if SOC>=80
    Ibmax = Imax;
    Ibmin = Imin;
elseif SOC<80 && SOC>=20
    Ibmax = Imax;
    Ibmin = -Imax;
elseif SOC<20
    Ibmax = -Imin;
    Ibmin = -Imax;
end
